simulink model "FSPDiscreteSimulink"  (R2023b)
settings: Solver=VariableStepAuto  StartTime=0.0  StopTime=Tsim  RelTol=1e-3
values from neighbouring files (symbols this model uses):
  finaldisturbancevalue = 0.2    [FSPDiscrete.m]
  hd = h/Ts    (= 26)    [FSPDiscrete.m]
  initialdisturbancevalue = 0    [FSPDiscrete.m]
  Tdisturbance = 10    [FSPDiscrete.m]
  Ts = 0.25    [FSPDiscrete.m]
libraries: cstblocks x11
settings Model: Creator=klysm  LastModifiedBy=klysm

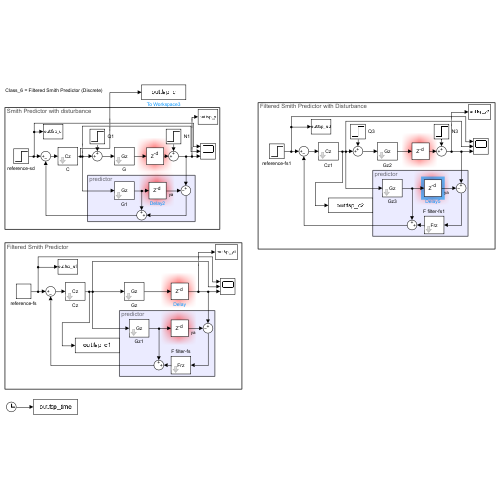
[thumbnail: Simulink's stored preview of the top-level diagram]
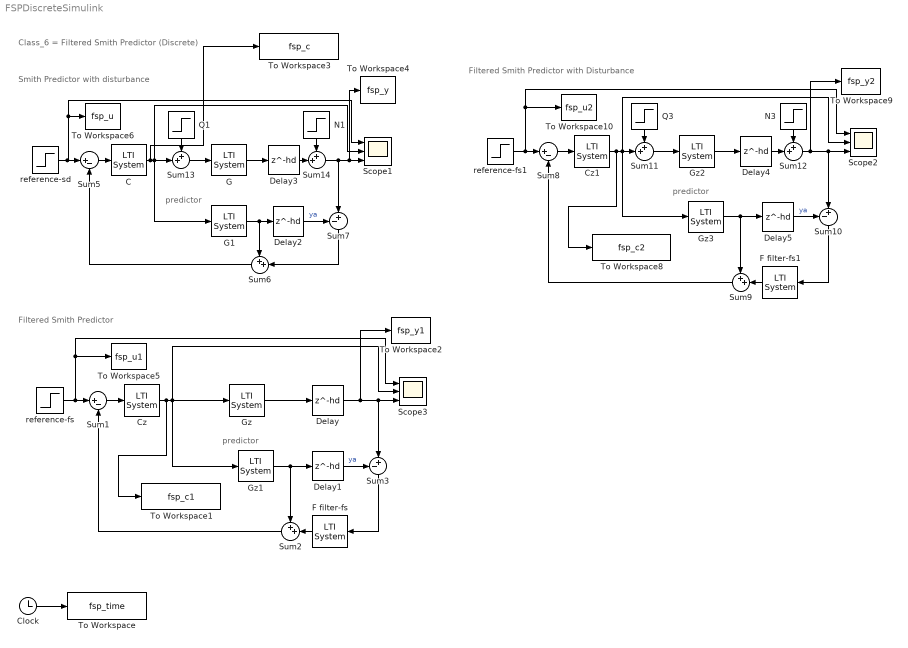
== system FSPDiscreteSimulink ==
  note: Class_6 = Filtered Smith Predictor (Discrete)
  note: Filtered Smith Predictor
  note: predictor
  note: predictor
  note: Smith Predictor with disturbance
  note: Filtered Smith Predictor with Disturbance
  note: predictor
  C : cstblocks/LTI System  sys=Cz  IC=[]  PadeOrder=0
  Clock : Clock
  Cz : cstblocks/LTI System  sys=Cz  IC=[]  PadeOrder=0
  Cz1 : cstblocks/LTI System  sys=Cz  IC=[]  PadeOrder=0
  Delay{,1..5} (6 alike) : Delay  DelayLength=hd  SampleTime=Ts
  F filter-fs : cstblocks/LTI System  sys=Frz  IC=[]  PadeOrder=0
  F filter-fs1 : cstblocks/LTI System  sys=Frz  IC=[]  PadeOrder=0
  G : cstblocks/LTI System  sys=Gz  IC=[]  PadeOrder=0
  G1 : cstblocks/LTI System  sys=Gz  IC=[]  PadeOrder=0
  Gz{,1..3} (4 alike) : cstblocks/LTI System  sys=Gz  IC=[]  PadeOrder=0
  N1 : Step  Time=20  Before=initialdisturbancevalue  After=finaldisturbancevalue  SampleTime=Ts
  N3 : Step  Time=20  Before=initialdisturbancevalue  After=finaldisturbancevalue  SampleTime=Ts
  Q1 : Step  Time=Tdisturbance  Before=initialdisturbancevalue  After=finaldisturbancevalue  SampleTime=Ts
  Q3 : Step  Time=Tdisturbance  Before=initialdisturbancevalue  After=finaldisturbancevalue  SampleTime=Ts
  Scope1 : Scope  NumInputPorts=3
  Scope2 : Scope  NumInputPorts=3
  Scope3 : Scope  NumInputPorts=3
  Sum1 : Sum  Inputs=|+-
  Sum10 : Sum  Inputs=-+|
  Sum{2,6,9,11..14} (7 alike) : Sum  Inputs=++|
  Sum3 : Sum  Inputs=-+|
  Sum5 : Sum  Inputs=|+-
  Sum7 : Sum  Inputs=-+|
  Sum8 : Sum  Inputs=|+-
  To Workspace : ToWorkspace  VariableName=fsp_time  SampleTime=Ts
  To Workspace1 : ToWorkspace  VariableName=fsp_c1  SampleTime=Ts
  To Workspace10 : ToWorkspace  VariableName=fsp_u2  SampleTime=Ts
  To Workspace2 : ToWorkspace  VariableName=fsp_y1  SampleTime=Ts
  To Workspace3 : ToWorkspace  VariableName=fsp_c  SampleTime=Ts
  To Workspace4 : ToWorkspace  VariableName=fsp_y  SampleTime=Ts
  To Workspace5 : ToWorkspace  VariableName=fsp_u1  SampleTime=Ts
  To Workspace6 : ToWorkspace  VariableName=fsp_u  SampleTime=Ts
  To Workspace8 : ToWorkspace  VariableName=fsp_c2  SampleTime=Ts
  To Workspace9 : ToWorkspace  VariableName=fsp_y2  SampleTime=Ts
  reference-fs : Step  Time=0  SampleTime=Ts
  reference-fs1 : Step  Time=0  SampleTime=Ts
  reference-sd : Step  Time=0  SampleTime=Ts
  wires:
  Sum3/1 -> F filter-fs/1
  reference-fs/1 -> To Workspace5/1, Scope3/1, Sum1/1
  Gz1/1 -> Delay1/1, Sum2/1
  Gz/1 -> Delay/1
  Sum2/1 -> Sum1/2
  Delay1/1 -> Sum3/1  "ya"
  Cz/1 -> To Workspace1/1, Gz/1, Gz1/1, Scope3/2
  Delay/1 -> Scope3/3, Sum3/2, To Workspace2/1
  Sum1/1 -> Cz/1
  F filter-fs/1 -> Sum2/2
  Q1/1 -> Sum13/1
  Sum13/1 -> G/1
  Sum5/1 -> C/1
  Sum14/1 -> To Workspace4/1, Scope1/3, Sum7/2
  Delay2/1 -> Sum7/1  "ya"
  G1/1 -> Delay2/1, Sum6/1
  Sum6/1 -> Sum5/2
  Sum7/1 -> Sum6/2
  reference-sd/1 -> To Workspace6/1, Scope1/1, Sum5/1
  G/1 -> Delay3/1
  C/1 -> To Workspace3/1, G1/1, Sum13/2, Scope1/2
  Clock/1 -> To Workspace/1
  Sum10/1 -> F filter-fs1/1
  Q3/1 -> Sum11/1
  Delay5/1 -> Sum10/1  "ya"
  Sum11/1 -> Gz2/1
  Sum9/1 -> Sum8/2
  Cz1/1 -> To Workspace8/1, Gz3/1, Scope2/2, Sum11/2
  Gz2/1 -> Delay4/1
  Sum8/1 -> Cz1/1
  Sum12/1 -> To Workspace9/1, Scope2/3, Sum10/2
  reference-fs1/1 -> To Workspace10/1, Scope2/1, Sum8/1
  F filter-fs1/1 -> Sum9/2
  Gz3/1 -> Delay5/1, Sum9/1
  Delay4/1 -> Sum12/2
  N3/1 -> Sum12/1
  Delay3/1 -> Sum14/2
  N1/1 -> Sum14/1
